simulink model "slave_task"  (Simulink 3.00)
libraries: inoutlib x4, mathlib x3

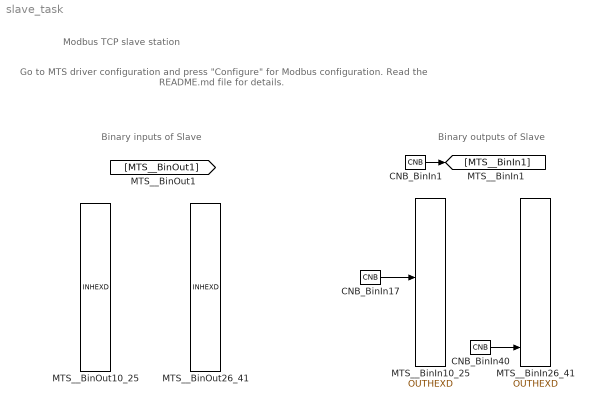
== system slave_task ==
  note: Binary inputs of Slave
  note: Binary outputs of Slave
  note: Modbus TCP slave station
  note: Go to MTS driver configuration and press "Configure" for Modbus configuration.
      |
      | Read the README.md file for details.
  CNB_BinIn1 : mathlib/CNB  YCN=off
  CNB_BinIn17 : mathlib/CNB  YCN=on
  CNB_BinIn40 : mathlib/CNB  YCN=on
  MTS__BinIn10_25 : inoutlib/OUTHEXD
  MTS__BinIn26_41 : inoutlib/OUTHEXD
  MTS__BinOut10_25 : inoutlib/INHEXD
  MTS__BinOut26_41 : inoutlib/INHEXD
  wires:
  CNB_BinIn1/1 -> [MTS__BinIn1]
  CNB_BinIn17/1 -> MTS__BinIn10_25/8
  CNB_BinIn40/1 -> MTS__BinIn26_41/15
